simulink model "HybridSaccadeFF"  (R2020a)
settings: Solver=FixedStepAuto  StartTime=0  StopTime=5  FixedStep=0.001  RelTol=1e-3
undefined symbols (not defined in the file): K_I, K_P, n_delay, sac_time, switch_thresh, T_lim_low, T_lim_up
libraries: cstblocks x1
settings Model: PacingRate=0.010000  Creator=Brock  LastModifiedBy=Brock

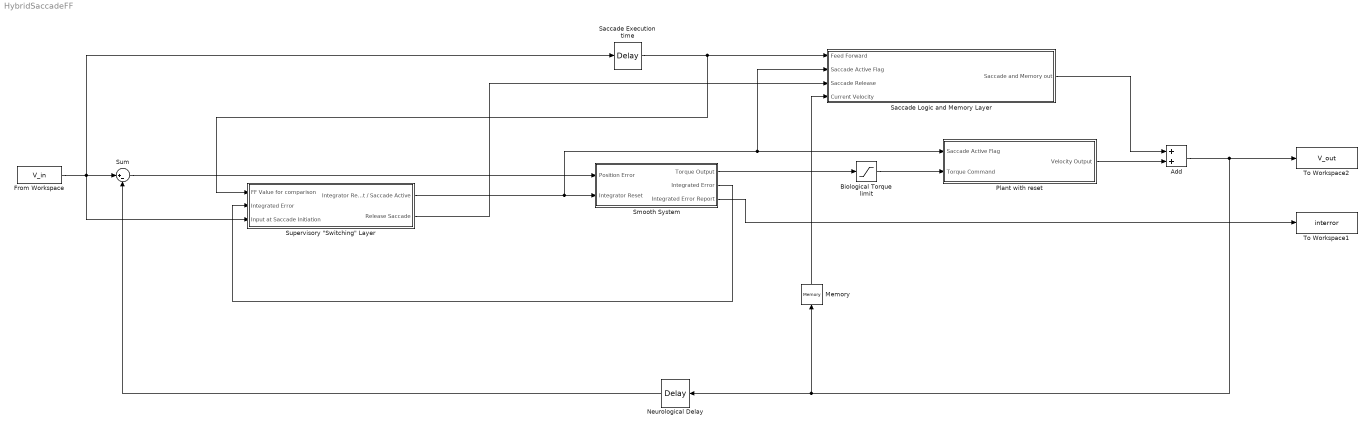
== system HybridSaccadeFF ==
  Add : Sum
  Biological Torque limit : Saturate  UpperLimit=T_lim_up  LowerLimit=T_lim_low  LinearizeAsGain=off
  From Workspace : FromWorkspace  VariableName=V_in
  Memory : Memory
  Neurological Delay : TransportDelay  DelayTime=n_delay
  Plant with reset : Subsystem
  Saccade Execution time : TransportDelay  DelayTime=sac_time
  Saccade Logic and Memory Layer : Subsystem
  Smooth System : Subsystem
  Sum : Sum  Inputs=|+-
  "Supervisory \"Switching\" Layer" : Subsystem
  To Workspace1 : ToWorkspace  VariableName=interror  SampleTime=-1
  To Workspace2 : ToWorkspace  VariableName=V_out  SampleTime=-1
  wires:
  Add/1 -> To Workspace2/1, Neurological Delay/1, Memory/1
  Smooth System/1(Torque Output) -> Biological Torque limit/1
  Saccade Execution time/1 -> "Supervisory \"Switching\" Layer"/1(FF Value for comparison), Saccade Logic and Memory Layer/1(Feed Forward)
  Smooth System/2(Integrated Error) -> "Supervisory \"Switching\" Layer"/2(Integrated Error)
  Sum/1 -> Smooth System/1(Position Error)
  From Workspace/1 -> "Supervisory \"Switching\" Layer"/3(Input at Saccade Initiation), Saccade Execution time/1, Sum/1
  "Supervisory \"Switching\" Layer"/2(Release Saccade) -> Saccade Logic and Memory Layer/3(Saccade Release)
  Saccade Logic and Memory Layer/1(Saccade and Memory out) -> Add/1
  Biological Torque limit/1 -> Plant with reset/2(Torque Command)
  Plant with reset/1(Velocity Output) -> Add/2
  Smooth System/3(Integrated Error Report) -> To Workspace1/1
  Memory/1 -> Saccade Logic and Memory Layer/4(Current Velocity)
  Neurological Delay/1 -> Sum/2
  "Supervisory \"Switching\" Layer"/1(Integrator Reset / Saccade Active) -> Saccade Logic and Memory Layer/2(Saccade Active Flag), Plant with reset/1(Saccade Active Flag), Smooth System/2(Integrator Reset)

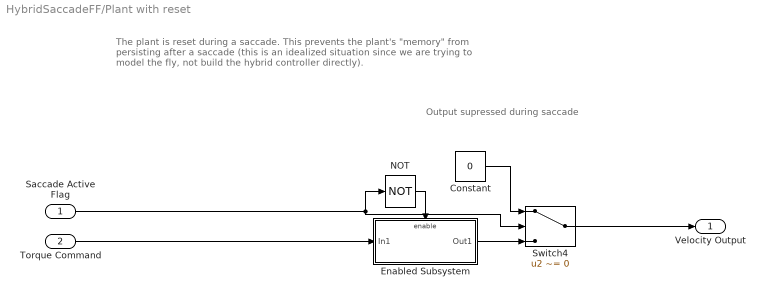
== system HybridSaccadeFF/Plant with reset ==
  note: The plant is reset during a saccade.  This prevents the plant's "memory"
      | from persisting after a saccade (this is an idealized situation since we are
      | trying to model the fly, not build the hybrid controller directly).
  note: Output supressed during saccade
  Saccade Active Flag : Inport
  Torque Command : Inport  Port=2
  Constant : Constant  Value=0
  Enabled Subsystem : Subsystem  TreatAsAtomicUnit=on
  NOT : Logic  Operator=NOT  IconShape=distinctive  AllPortsSameDT=off  OutDataTypeStr=boolean
  Switch4 : Switch  Criteria=u2 ~= 0
  Velocity Output : Outport
  wires:
  Constant/1 -> Switch4/1
  NOT/1 -> Enabled Subsystem/Enable
  Enabled Subsystem/1(Out1) -> Switch4/3
  Saccade Active Flag/1 -> Switch4/2, NOT/1
  Switch4/1 -> Velocity Output/1
  Torque Command/1 -> Enabled Subsystem/1(In1)

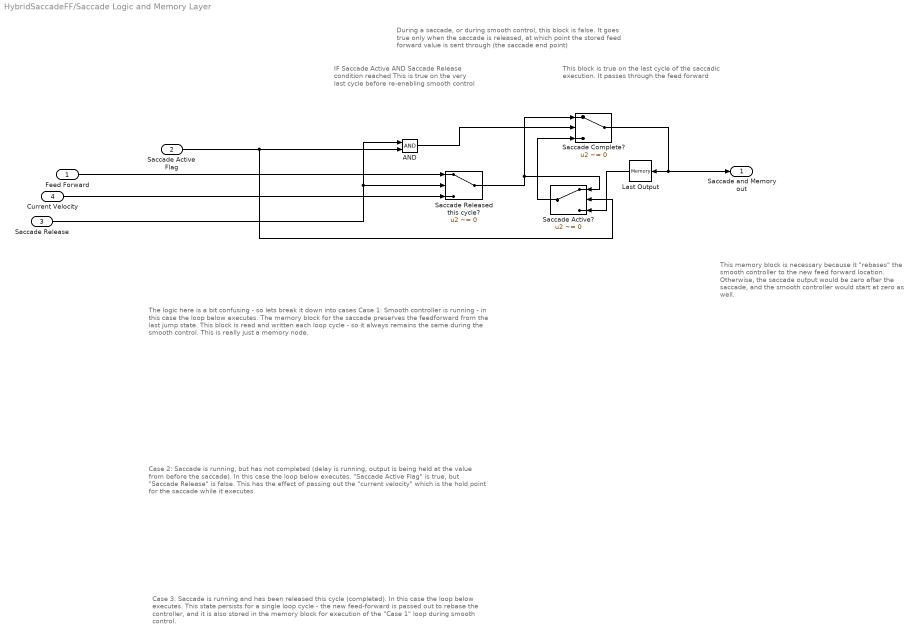
== system HybridSaccadeFF/Saccade Logic and Memory Layer ==
  note: The logic here is a bit confusing - so lets break it down into cases
      | Case 1: Smooth controller is running - in this case the loop below executes.  The memory block for the saccade preserves the feedforward from the last jump state.
      | This block is read and written each loop cycle - so it always remains the same during the smooth control.  This is really just a memory node.
  note: IF Saccade Active
      | AND Saccade Release condition reached
      | This is true on the very last cycle before
      | re-enabling smooth control
  note: During a saccade, or during smooth control, this block is false.
      | It goes true only when the saccade is released, at which point the
      | stored feed forward value is sent through (the saccade end point)
  note: This block is true on the last cycle of the saccadic
      | execution.  It passes through the feed forward
  note: This memory block is necessary because it
      | "rebases" the smooth controller to the new feed
      | forward location.  Otherwise, the saccade output would
      | be zero after the saccade, and the smooth controller
      | would start at zero as well.
  note: Case 2: Saccade is running, but has not completed (delay is running, output is being held at the value from before the saccade).  In this case the loop below executes.
      | "Saccade Active Flag" is true, but "Saccade Release" is false.  This has the effect of passing out the "current velocity" which is the hold point for the saccade while it executes.
  note: Case 3: Saccade is running and has been released this cycle (completed).  In this case the loop below executes.
      | This state persists for a single loop cycle - the new feed-forward is passed out to rebase the controller, and it is also stored in the memory block for execution of the "Case 1"
      | loop during smooth control.
  Feed Forward : Inport
  Saccade Active Flag : Inport  Port=2
  Saccade Release : Inport  Port=3
  Current Velocity : Inport  Port=4
  AND : Logic  IconShape=distinctive  AllPortsSameDT=off  OutDataTypeStr=boolean
  Last Output : Memory
  Saccade Active? : Switch  Criteria=u2 ~= 0
  Saccade Complete? : Switch  Criteria=u2 ~= 0
  Saccade Released this cycle? : Switch  Criteria=u2 ~= 0
  Saccade and Memory out : Outport
  wires:
  Saccade Active?/1 -> Saccade Complete?/3
  Saccade Release/1 -> AND/1, Saccade Released this cycle?/2
  Saccade Released this cycle?/1 -> Saccade Active?/1, Saccade Complete?/1
  Saccade Complete?/1 -> Saccade and Memory out/1, Last Output/1
  Feed Forward/1 -> Saccade Released this cycle?/1
  Last Output/1 -> Saccade Active?/3
  Saccade Active Flag/1 -> Saccade Active?/2, AND/2
  Current Velocity/1 -> Saccade Released this cycle?/3
  AND/1 -> Saccade Complete?/2

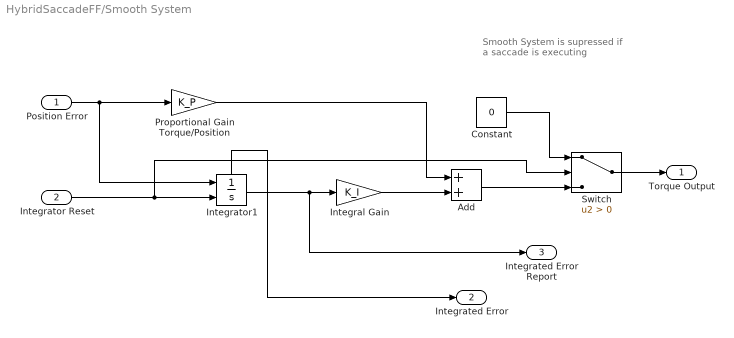
== system HybridSaccadeFF/Smooth System ==
  note: Smooth System is supressed
      | if a saccade is executing
  Position Error : Inport
  Integrator Reset : Inport  Port=2
  Add : Sum
  Constant : Constant  Value=0
  "Integral Gain " : Gain  Gain=K_I
  Integrator1 : Integrator  ExternalReset=level hold  ShowStatePort=on
  Proportional Gain Torque/Position : Gain  Gain=K_P
  Switch : Switch  Criteria=u2 > Threshold
  Torque Output : Outport
  Integrated Error : Outport  Port=2
  Integrated Error Report : Outport  Port=3
  wires:
  Proportional Gain Torque/Position/1 -> Add/1
  Integrator Reset/1 -> Switch/2, Integrator1/2
  Position Error/1 -> Integrator1/1, Proportional Gain Torque/Position/1
  Integrator1/State -> Integrated Error/1
  Integrator1/1 -> Integrated Error Report/1, "Integral Gain "/1
  "Integral Gain "/1 -> Add/2
  Add/1 -> Switch/3
  Switch/1 -> Torque Output/1
  Constant/1 -> Switch/1

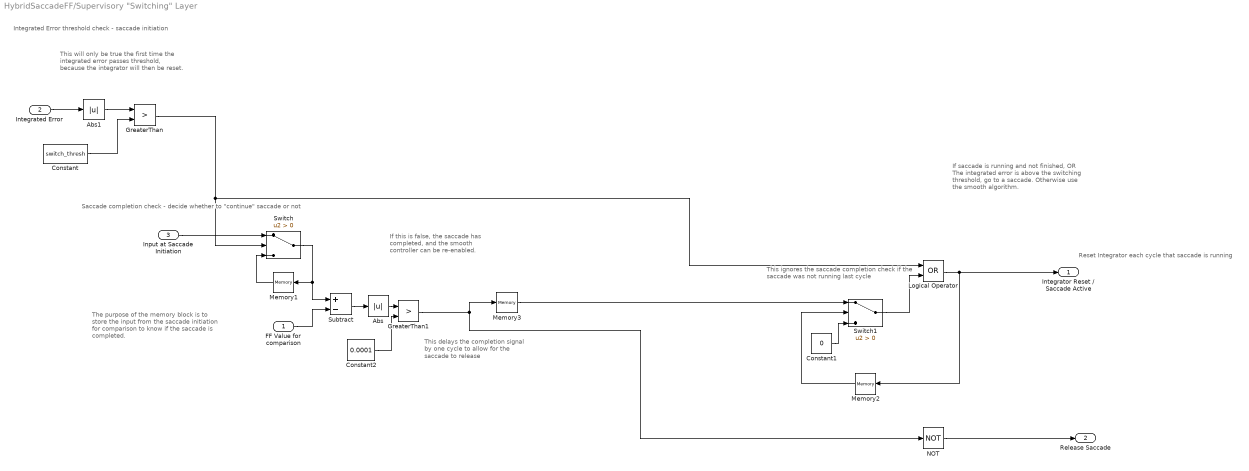
== system HybridSaccadeFF/Supervisory "Switching" Layer ==
  note: This ignores the saccade completion
      | check if the saccade was not running
      | last cycle
  note: Saccade completion check - decide whether to "continue" saccade or not
  note: Integrated Error threshold check - saccade initiation
  note: If saccade is running and not finished,
      | OR
      | The integrated error is above the switching threshold, go to a saccade.
      | Otherwise use the smooth algorithm.
  note: Reset Integrator each cycle that saccade is running
  note: This will only be true the first time the integrated error passes threshold, because the integrator will then be reset.
  note: If this is false, the saccade has completed, and the smooth controller can be re-enabled.
  note: The purpose of the memory block is to store the input from the saccade initiation for comparison to know if the saccade is completed.
  note: This delays the completion signal by one cycle to allow for the saccade to release
  FF Value for comparison : Inport
  Integrated Error : Inport  Port=2
  Input at Saccade Initiation : Inport  Port=3
  Abs : Abs
  Abs1 : Abs
  Constant : Constant  Value=switch_thresh
  Constant1 : Constant  Value=0
  Constant2 : Constant  Value=0.0001
  GreaterThan : RelationalOperator  Operator=>  OutDataTypeStr=boolean  RndMeth=Simplest
  GreaterThan1 : RelationalOperator  Operator=>  OutDataTypeStr=boolean  RndMeth=Simplest
  Logical Operator : Logic  Operator=OR  AllPortsSameDT=off  OutDataTypeStr=boolean
  Memory1 : Memory
  Memory2 : Memory
  Memory3 : Memory
  NOT : Logic  Operator=NOT  IconShape=distinctive  AllPortsSameDT=off  OutDataTypeStr=boolean
  Subtract : Sum  Inputs=+-
  Switch : Switch  Criteria=u2 > Threshold
  Switch1 : Switch  Criteria=u2 > Threshold
  Integrator Reset / Saccade Active : Outport
  Release Saccade : Outport  Port=2
  wires:
  Constant/1 -> GreaterThan/2
  GreaterThan/1 -> Logical Operator/1, Switch/2
  Logical Operator/1 -> Integrator Reset / Saccade Active/1, Memory2/1
  Input at Saccade Initiation/1 -> Switch/1
  Switch/1 -> Subtract/1, Memory1/1
  Memory1/1 -> Switch/3
  Memory2/1 -> Switch1/2
  GreaterThan1/1 -> Memory3/1, NOT/1
  Constant1/1 -> Switch1/3
  Switch1/1 -> Logical Operator/2
  Memory3/1 -> Switch1/1
  NOT/1 -> Release Saccade/1
  Subtract/1 -> Abs/1
  FF Value for comparison/1 -> Subtract/2
  Abs/1 -> GreaterThan1/1
  Constant2/1 -> GreaterThan1/2
  Abs1/1 -> GreaterThan/1
  Integrated Error/1 -> Abs1/1

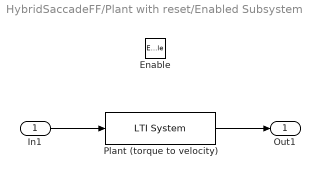
== system HybridSaccadeFF/Plant with reset/Enabled Subsystem ==
  In1 : Inport
  Enable : EnablePort  StatesWhenEnabling=reset
  Plant (torque to velocity) : cstblocks/LTI System  sys=G_plant  IC=[]
  Out1 : Outport
  wires:
  Plant (torque to velocity)/1 -> Out1/1
  In1/1 -> Plant (torque to velocity)/1
